simulink model "kp_j_inv"  (R2021a)
settings: Solver=VariableStepAuto  StartTime=0.0  StopTime=100  RelTol=1e-3
values from neighbouring files (symbols this model uses):
  k = [1 1;1 1;1 1]    [eval_mod.m]    (also in sim_q3.m = 1)
  kp = (f/z0)*[alfa 0; 0 alfa]*[cos(phi) sin(phi); sin(phi) -cos(phi)]    [mdl_planar_2r.m]
  kp2 = (f/z0)*[alfa 0; 0 alfa]*[cos(phi2) sin(phi2); sin(phi2) -cos(phi2)]    [mdl_planar_2r.m]
  q0 = [0, 15, 180, -130, 0, 55, 90]    [mdl_kinovagen3_trab2.m]    (also in mdl_planar_2r.m = [-pi/20, -pi/2])
  wn = 2*pi/10    (= 0.628318530718)    [eval_mod.m]    (also in mdl_planar_2r.m = 1)
  xco2 = (f/z0)*[alfa 0; 0 alfa]*[-cos(phi2) -sin(phi2);-sin(phi2) cos(phi2)]*p_bc + oc    [mdl_planar_2r.m]
libraries: roblocks x3, simulink x2
settings Model: Creator=Guga  LastModifiedBy=Guga

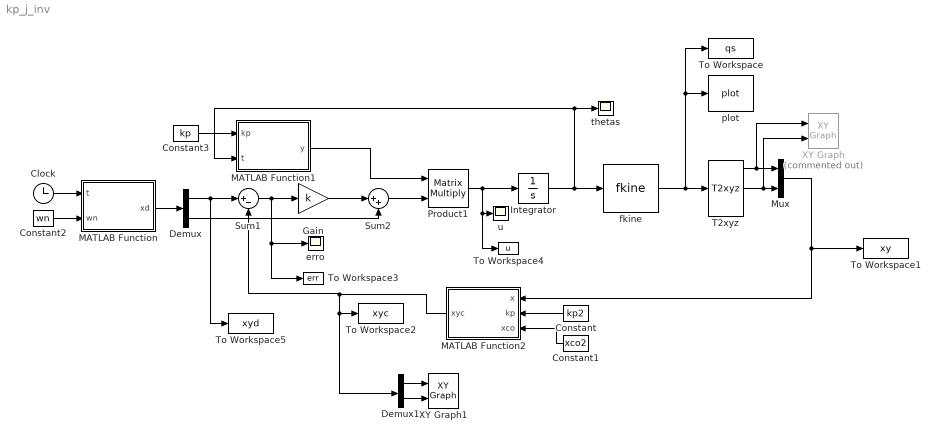
== system kp_j_inv ==
  Clock : Clock
  Constant : Constant  Value=kp2
  Constant1 : Constant  Value=xco2
  Constant2 : Constant  Value=wn
  Constant3 : Constant  Value=kp
  Demux : Demux  Outputs=2
  Demux1 : Demux  Outputs=2
  Gain : Gain  Gain=k
  Integrator : Integrator  InitialCondition=q0
  MATLAB Function : MATLAB Function  TreatAsAtomicUnit=on
  MATLAB Function1 : MATLAB Function  TreatAsAtomicUnit=on
  MATLAB Function2 : MATLAB Function  TreatAsAtomicUnit=on
  Mux : Mux  Inputs=2
  Product1 : Product  Multiplication=Matrix(*)
  Sum1 : Sum  Inputs=|+-
  Sum2 : Sum  Inputs=|++
  T2xyz : roblocks/Toolbox/T2xyz
  To Workspace : ToWorkspace  VariableName=qs  SaveFormat=Timeseries  SampleTime=-1
  To Workspace1 : ToWorkspace  VariableName=xy  SaveFormat=Timeseries  SampleTime=-1
  To Workspace2 : ToWorkspace  VariableName=xyc  SaveFormat=Timeseries  SampleTime=-1
  To Workspace3 : ToWorkspace  VariableName=err  SaveFormat=Timeseries  SampleTime=-1
  To Workspace4 : ToWorkspace  VariableName=u  SaveFormat=Timeseries  SampleTime=-1
  To Workspace5 : ToWorkspace  VariableName=xyd  SaveFormat=Timeseries  SampleTime=-1
  XY Graph : simulink/Sinks/XY Graph  Commented=on  xmin=-1  xmax=1  ymin=-1  ymax=1  st=-1
  XY Graph1 : simulink/Sinks/XY Graph  xmin=0  xmax=500  ymin=0  ymax=500  st=-1
  erro : Scope
  fkine : roblocks/Arm/fkine  robot=planar2r
  plot : roblocks/Arm/plot  robot=planar2r  fps=5  holdplot=on
  thetas : Scope
  u : Scope
  wires:
  Clock/1 -> MATLAB Function/1(t)
  MATLAB Function/1(xd) -> Demux/1
  MATLAB Function2/1(xyc) -> Demux1/1, To Workspace2/1, Sum1/2
  Sum1/1 -> To Workspace3/1, erro/1, Gain/1
  Gain/1 -> Sum2/1
  Demux/1 -> To Workspace5/1, Sum1/1
  Demux/2 -> Sum2/2
  Sum2/1 -> Product1/2
  MATLAB Function1/1(y) -> Product1/1
  fkine/1 -> To Workspace/1, plot/1, T2xyz/1
  T2xyz/1 -> XY Graph/1, Mux/1
  T2xyz/2 -> XY Graph/2, Mux/2
  Integrator/1 -> thetas/1, MATLAB Function1/2(t), fkine/1
  Constant2/1 -> MATLAB Function/2(wn)
  Product1/1 -> To Workspace4/1, u/1, Integrator/1
  Mux/1 -> To Workspace1/1, MATLAB Function2/1(x)
  Constant/1 -> MATLAB Function2/2(kp)
  Constant1/1 -> MATLAB Function2/3(xco)
  Demux1/2 -> XY Graph1/2
  Demux1/1 -> XY Graph1/1
  Constant3/1 -> MATLAB Function1/1(kp)

== matlab function kp_j_inv/MATLAB Function1 ==
  data: kp input; y output; t input
function y = fcn(kp,t)
d1 = 0.42;
d2 = 0.31;
ja = [-d1*sin(t(1))-d2*sin(t(1)+t(2)) -d2*sin(t(1)+t(2));d1*cos(t(1))+d2*cos(t(1)+t(2)) d2*cos(t(1)+t(2))];
y = pinv(kp*ja);

end

== matlab function kp_j_inv/MATLAB Function ==
  data: t input; xd output; wn input
function xd = fcn(t,wn)

xd = [300+60*(sin(wn*t)+sin(1.5*wn*t));
    200+60*(sin(wn*t+1.6)+sin(1.5*wn*t+1.6));
    60*(wn*cos(wn*t)+1.5*wn*cos(1.5*wn*t));
    60*(wn*cos(wn*t+1.6)+1.5*wn*cos(1.5*wn*t+1.6))];
end

== matlab function kp_j_inv/MATLAB Function2 ==
  data: x input; kp input; xyc output; xco input
function xyc = fcn(x,kp,xco)

xyc = kp*x+xco;

end
